simulink model "spacecraft_using_vertices_and_faces"  (R2018b)
settings: Solver=ode4  StartTime=0.0  StopTime=60000  FixedStep=0.1  RelTol=1e-3
libraries: simulink x6
settings Model: Creator=do  LastModifiedBy=do

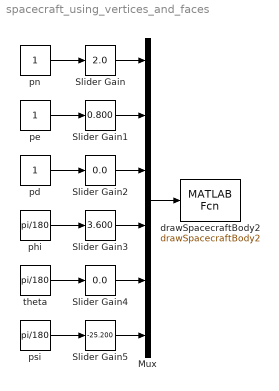
== system spacecraft_using_vertices_and_faces ==
  Mux : Mux  Inputs=6
  Slider Gain : simulink/Math Operations/Slider Gain  gain=2.0  low=-10  high=10
  Slider Gain1 : simulink/Math Operations/Slider Gain  gain=0.800  low=-10  high=10
  Slider Gain2 : simulink/Math Operations/Slider Gain  gain=0.0  low=-180  high=180
  Slider Gain3 : simulink/Math Operations/Slider Gain  gain=3.600  low=-180  high=180
  Slider Gain4 : simulink/Math Operations/Slider Gain  gain=0.0  low=-180  high=180
  Slider Gain5 : simulink/Math Operations/Slider Gain  gain=-25.200  low=-180  high=180
  drawSpacecraftBody2 : MATLABFcn  MATLABFcn=drawSpacecraftBody2  OutputDimensions=0
      mask init:
      | XYZ = [...
      |     1       1       0;... % point 1
      |     1       -1      0;... % point 2
      |     -1      -1      0;... % point 3
      |     -1      1       0;... % point 4
      |     1       1       0;... % point 1
      |     1       1       -2;... % point 5
      |     1       -1      -2;... % point 6
      |     1       -1      0;... % point 2
      |     1       -1      -2;... % point 6
      |     -1      -1      -2;... % point 7
      |     -1      -1      0;... % point 3
      |     -1      -1      -2;... % point 7
      |     -1      1       -2;... % point 8
      |     -1       1       0;... % point 4
      |     -1      1       -2;... % point 8
      |     1       1       -2;... % point 5
      |     1       1       0;... % point 1
      |     1.5     1.5    0;... % point 9
      |     1.5     -1.5   0;... % point 10
      |     1       -1      0;... % point 2
      |     1.5     -1.5   0;... % point 10
      |     -1.5    -1.5   0;... % point 11
      |     -1      -1      0;... % point 3
      |     -1.5    -1.5   0;... % point 11
      |     -1.5    1.5    0;... % point 12
      |     -1      1       0;... % point 4
      |     -1.5    1.5    0;... % point 12
      |     1.5     1.5     0;... % point 9
      | ]';
  pd : Constant
  pe : Constant
  phi : Constant  Value=pi/180
  "pn " : Constant
  psi : Constant  Value=pi/180
  theta : Constant  Value=pi/180
  wires:
  "pn "/1 -> Slider Gain/1
  pe/1 -> Slider Gain1/1
  pd/1 -> Slider Gain2/1
  phi/1 -> Slider Gain3/1
  theta/1 -> Slider Gain4/1
  psi/1 -> Slider Gain5/1
  Mux/1 -> drawSpacecraftBody2/1
  Slider Gain/1 -> Mux/1
  Slider Gain1/1 -> Mux/2
  Slider Gain2/1 -> Mux/3
  Slider Gain3/1 -> Mux/4
  Slider Gain4/1 -> Mux/5
  Slider Gain5/1 -> Mux/6
